simulink library "sofar"  (R2017a)
settings: Solver=VariableStepAuto  StartTime=0.0  StopTime=10.0  RelTol=1e-3
settings Model: Creator=mudat  LastModifiedBy=mudat

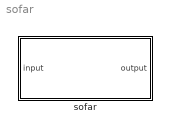
== system sofar ==
  sofar : Subsystem

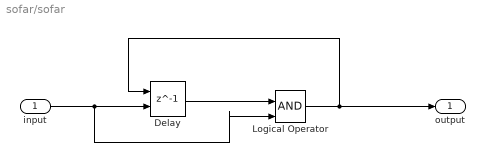
== system sofar/sofar ==
  input : Inport  OutDataTypeStr=boolean
  Delay : Delay  DelayLength=1  InitialConditionSource=Input port
      settings: InputPortMap=u0,p4
  Logical Operator : Logic  IconShape=distinctive  AllPortsSameDT=off  OutDataTypeStr=boolean
  output : Outport
  wires:
  Logical Operator/1 -> output/1, Delay/1
  Delay/1 -> Logical Operator/1
  input/1 -> Logical Operator/2, Delay/2
